simulink model "obstacle"  (R2017a)
settings: Solver=VariableStepAuto  StartTime=0.0  StopTime=10  FixedStep=0.05  RelTol=1e-3
values from neighbouring files (symbols this model uses):
  distance_of_CG = vehical_length/2    (= 0.1825)    [init.m]
  o_x1 = 3    [init.m]
  o_x2 = 5    [init.m]
  o_y1 = 3.3    [init.m]
  o_y2 = 4.7    [init.m]
  psi_init = deg2rad(45)    [init.m]
  x_init = 0    [init.m]
  y_init = 0.2    [init.m]
undefined symbols (not defined in the file or in its folder): theta, x0, y0
undefined symbols (not defined in the file): vehical_length
libraries: simulink_extras x2, simulink x1
settings Model: SnapshotInterval=1  Creator=dell  LastModifiedBy=dell
settings DebuggingCC: InheritedTsInSrcMsg=error

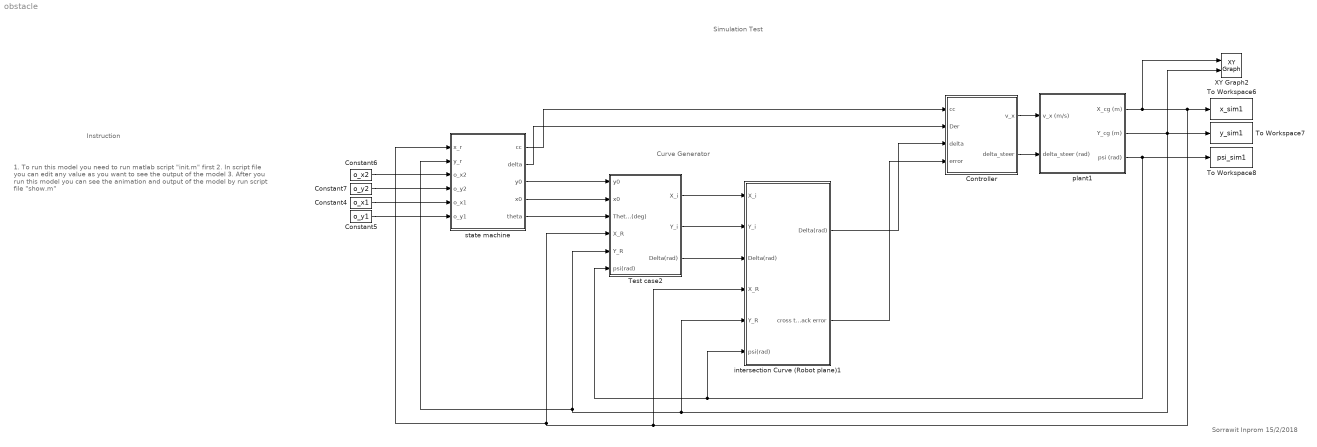
== system obstacle ==
  note: Simulation Test
  note: Sorrawit Inprom
      | 15/2/2018
  note: Curve Generator
  note: Instruction
  note: 1. To run this model you need to run matlab script "init.m" first
      |
      | 2. In script file you can edit any value as you want to see the output of the model
      |
      | 3. After you run this model you can see the animation and output of the model by run script file "show.m"
  Constant4 : Constant  Value=o_x1
  Constant5 : Constant  Value=o_y1
  Constant6 : Constant  Value=o_x2
  Constant7 : Constant  Value=o_y2
  Controller : Subsystem
  Test case2 : Subsystem
  To Workspace6 : ToWorkspace  VariableName=x_sim1  SaveFormat=Timeseries  SampleTime=-1
  To Workspace7 : ToWorkspace  VariableName=y_sim1  SaveFormat=Timeseries  SampleTime=-1
  To Workspace8 : ToWorkspace  VariableName=psi_sim1  SaveFormat=Timeseries  SampleTime=-1
  XY Graph2 : simulink/Sinks/XY Graph  xmin=0  xmax=10  ymin=-1  ymax=10  st=-1
  intersection Curve (Robot plane)1 : Subsystem
  plant1 : Subsystem  mask{vehicle_length=vehical_length, distance_of_CG=distance_of_CG}
      mask prompts: vehicle_length "length"; distance_of_CG "CG"
  state machine : Stateflow chart  TreatAsAtomicUnit=on
  wires:
  state machine/3(y0) -> Test case2/1(y0)
  state machine/4(x0) -> Test case2/2(x0)
  state machine/5(theta) -> Test case2/3(Theta(deg))
  Test case2/1(X_i) -> intersection Curve (Robot plane)1/1(X_i)
  Test case2/2(Y_i) -> intersection Curve (Robot plane)1/2(Y_i)
  Test case2/3("Delta(rad) ") -> intersection Curve (Robot plane)1/3(Delta(rad))
  intersection Curve (Robot plane)1/1("Delta(rad) ") -> Controller/3(delta)
  intersection Curve (Robot plane)1/2(cross track error) -> Controller/4(error)
  Controller/2(delta_steer) -> plant1/2(delta_steer (rad))
  Controller/1(v_x) -> plant1/1(v_x (m/s))
  state machine/1(cc) -> Controller/1(cc)
  state machine/2(delta) -> Controller/2(Der)
  plant1/1(X_cg (m)) -> To Workspace6/1, intersection Curve (Robot plane)1/4(X_R), state machine/1(x_r), Test case2/4(X_R), XY Graph2/1
  plant1/2(Y_cg (m)) -> intersection Curve (Robot plane)1/5(Y_R), state machine/2(y_r), Test case2/5(Y_R), To Workspace7/1, XY Graph2/2
  plant1/3(psi (rad)) -> intersection Curve (Robot plane)1/6(psi(rad)), Test case2/6(psi(rad)), To Workspace8/1
  Constant6/1 -> state machine/3(o_x2)
  Constant7/1 -> state machine/4(o_y2)
  Constant4/1 -> state machine/5(o_x1)
  Constant5/1 -> state machine/6(o_y1)

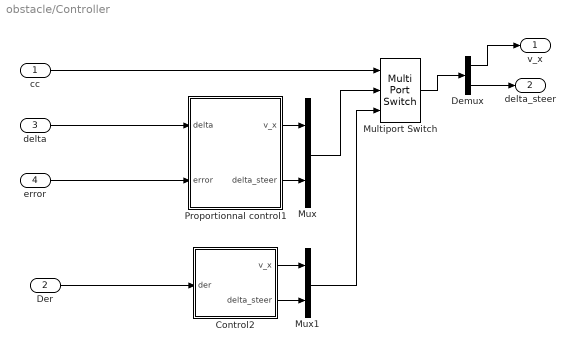
== system obstacle/Controller ==
  cc : Inport
  Der : Inport  Port=2
  delta : Inport  Port=3
  error : Inport  Port=4
  Control2 : Subsystem
  Demux : Demux  Outputs=2
  Multiport Switch : MultiPortSwitch  Inputs=2  DiagnosticForDefault=None
  Mux : Mux  Inputs=2
  Mux1 : Mux  Inputs=2
  Proportionnal control1 : Subsystem
  v_x : Outport
  delta_steer : Outport  Port=2
  wires:
  Multiport Switch/1 -> Demux/1
  Proportionnal control1/2(delta_steer) -> Mux/2
  Mux/1 -> Multiport Switch/2
  Demux/1 -> v_x/1
  Control2/1(v_x) -> Mux1/1
  error/1 -> Proportionnal control1/2(error)
  Der/1 -> Control2/1(der)
  delta/1 -> Proportionnal control1/1(delta)
  Mux1/1 -> Multiport Switch/3
  Control2/2(delta_steer) -> Mux1/2
  cc/1 -> Multiport Switch/1
  Proportionnal control1/1(v_x) -> Mux/1
  Demux/2 -> delta_steer/1

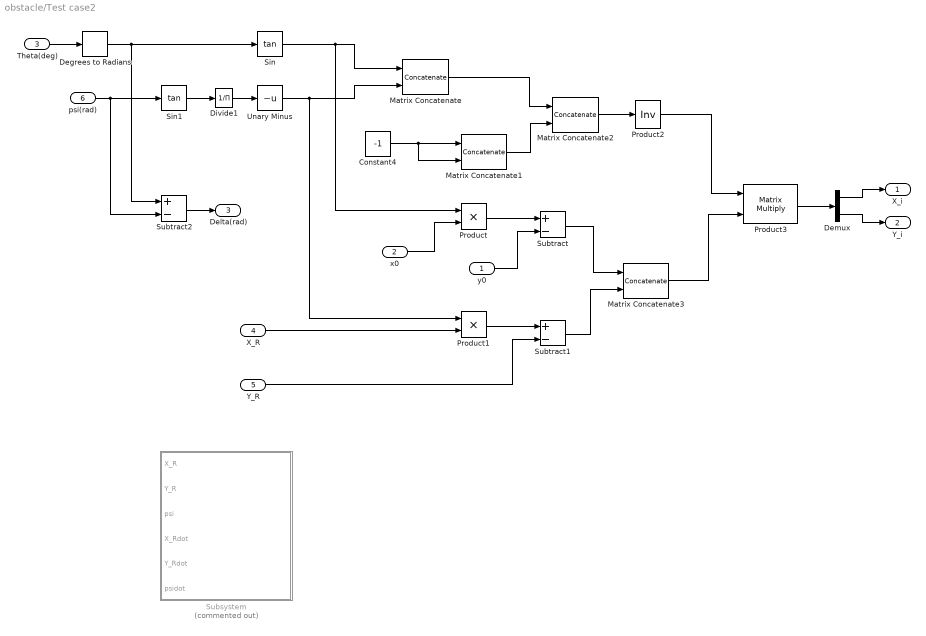
== system obstacle/Test case2 ==
  y0 : Inport
  x0 : Inport  Port=2
  Theta(deg) : Inport  Port=3
  X_R : Inport  Port=4
  Y_R : Inport  Port=5
  psi(rad) : Inport  Port=6
  Constant4 : Constant  Value=-1
  Degrees to Radians : simulink_extras/Transformations/Degrees to Radians
  Demux : Demux  Outputs=2
  Divide1 : Product  Inputs=/
  Matrix Concatenate : Concatenate  Mode=Multidimensional array
  Matrix Concatenate1 : Concatenate  Mode=Multidimensional array
  Matrix Concatenate2 : Concatenate  Mode=Multidimensional array  ConcatenateDimension=2
  Matrix Concatenate3 : Concatenate  Mode=Multidimensional array
  Product : Product
  Product1 : Product
  Product2 : Product  Inputs=/  Multiplication=Matrix(*)
  Product3 : Product  Multiplication=Matrix(*)
  Sin : Trigonometry  Operator=tan
  Sin1 : Trigonometry  Operator=tan
  Subsystem : Subsystem  Commented=on
  Subtract : Sum  Inputs=+-
  Subtract1 : Sum  Inputs=+-
  Subtract2 : Sum  Inputs=+-
  Unary Minus : UnaryMinus
  X_i : Outport
  Y_i : Outport  Port=2
  "Delta(rad) " : Outport  Port=3
  wires:
  Matrix Concatenate2/1 -> Product2/1
  X_R/1 -> Product1/2
  Demux/2 -> Y_i/1
  Matrix Concatenate3/1 -> Product3/2
  Divide1/1 -> Unary Minus/1
  Sin1/1 -> Divide1/1
  y0/1 -> Subtract/2
  x0/1 -> Product/2
  Demux/1 -> X_i/1
  Unary Minus/1 -> Product1/1, Matrix Concatenate/2
  Subtract/1 -> Matrix Concatenate3/1
  Y_R/1 -> Subtract1/2
  Product/1 -> Subtract/1
  Product1/1 -> Subtract1/1
  Subtract1/1 -> Matrix Concatenate3/2
  psi(rad)/1 -> Sin1/1, Subtract2/2
  Constant4/1 -> Matrix Concatenate1/2, Matrix Concatenate1/1
  Matrix Concatenate1/1 -> Matrix Concatenate2/2
  Product2/1 -> Product3/1
  Sin/1 -> Product/1, Matrix Concatenate/1
  Theta(deg)/1 -> Degrees to Radians/1
  Product3/1 -> Demux/1
  Subtract2/1 -> "Delta(rad) "/1
  Matrix Concatenate/1 -> Matrix Concatenate2/1
  Degrees to Radians/1 -> Sin/1, Subtract2/1

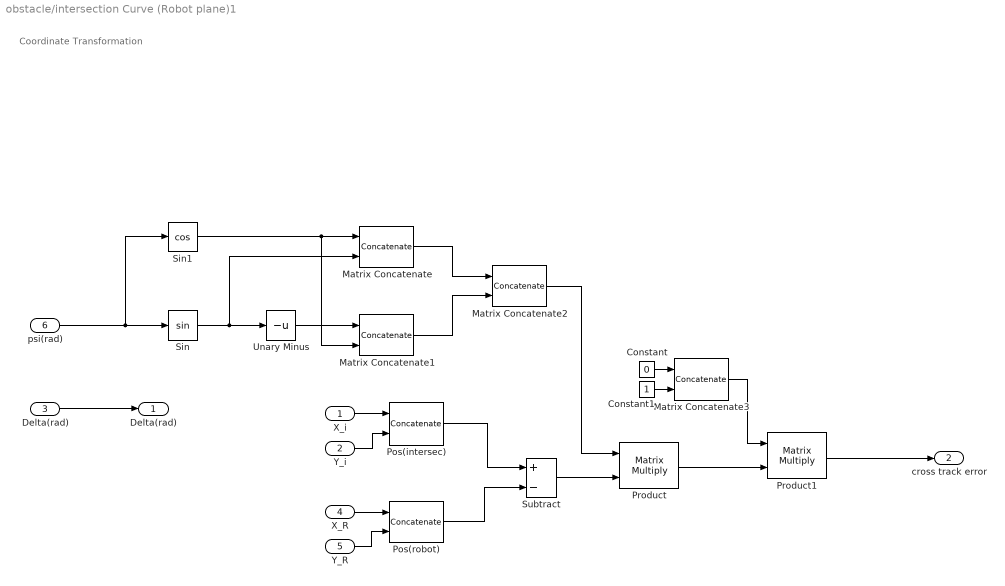
== system obstacle/intersection Curve (Robot plane)1 ==
  note: Coordinate Transformation
  X_i : Inport
  Y_i : Inport  Port=2
  Delta(rad) : Inport  Port=3
  X_R : Inport  Port=4
  Y_R : Inport  Port=5
  psi(rad) : Inport  Port=6
  Constant : Constant  Value=0
  Constant1 : Constant
  Matrix Concatenate : Concatenate  Mode=Multidimensional array  ConcatenateDimension=2
  Matrix Concatenate1 : Concatenate  Mode=Multidimensional array  ConcatenateDimension=2
  Matrix Concatenate2 : Concatenate  Mode=Multidimensional array
  Matrix Concatenate3 : Concatenate  Mode=Multidimensional array  ConcatenateDimension=2
  "Pos(intersec) " : Concatenate  Mode=Multidimensional array
  Pos(robot) : Concatenate  Mode=Multidimensional array
  Product : Product  Multiplication=Matrix(*)
  Product1 : Product  Multiplication=Matrix(*)
  Sin : Trigonometry
  Sin1 : Trigonometry  Operator=cos
  Subtract : Sum  Inputs=+-
  Unary Minus : UnaryMinus
  "Delta(rad) " : Outport
  cross track error : Outport  Port=2
  wires:
  psi(rad)/1 -> Sin1/1, Sin/1
  Matrix Concatenate2/1 -> Product/1
  X_i/1 -> "Pos(intersec) "/1
  Y_i/1 -> "Pos(intersec) "/2
  Subtract/1 -> Product/2
  "Pos(intersec) "/1 -> Subtract/1
  Pos(robot)/1 -> Subtract/2
  Unary Minus/1 -> Matrix Concatenate1/1
  Y_R/1 -> Pos(robot)/2
  X_R/1 -> Pos(robot)/1
  Matrix Concatenate1/1 -> Matrix Concatenate2/2
  Sin1/1 -> Matrix Concatenate/1, Matrix Concatenate1/2
  Matrix Concatenate/1 -> Matrix Concatenate2/1
  Sin/1 -> Matrix Concatenate/2, Unary Minus/1
  Delta(rad)/1 -> "Delta(rad) "/1
  Product/1 -> Product1/2
  Constant/1 -> Matrix Concatenate3/1
  Constant1/1 -> Matrix Concatenate3/2
  Matrix Concatenate3/1 -> Product1/1
  Product1/1 -> cross track error/1

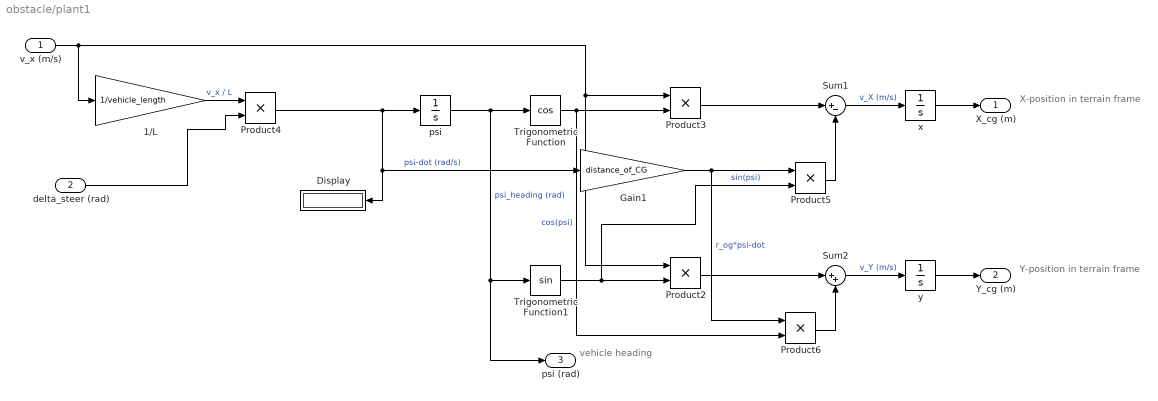
== system obstacle/plant1 ==
  note: vehicle
      | heading
  note: X-position in
      | terrain frame
  note: Y-position in
      | terrain frame
  v_x (m/s) : Inport
  delta_steer (rad) : Inport  Port=2
  1/L : Gain  Gain=1/vehicle_length
  Display : Display
  Gain1 : Gain  Gain=distance_of_CG
  Product{2..6} (5 alike) : Product  RndMeth=Zero
  Sum1 : Sum  Inputs=|+-
  Sum2 : Sum  Inputs=|++
  Trigonometric Function : Trigonometry  Operator=cos
  Trigonometric Function1 : Trigonometry
  psi : Integrator  InitialCondition=psi_init
  x : Integrator  InitialCondition=x_init
  y : Integrator  InitialCondition=y_init
  X_cg (m) : Outport
  Y_cg (m) : Outport  Port=2
  psi (rad) : Outport  Port=3
  wires:
  psi/1 -> Trigonometric Function/1, psi (rad)/1, Trigonometric Function1/1  "psi_heading (rad)"
  x/1 -> X_cg (m)/1
  Trigonometric Function/1 -> Product6/2, Product3/2  "cos(psi)"
  Product4/1 -> Gain1/1, Display/1, psi/1  "psi-dot (rad/s)"
  Sum2/1 -> y/1  "v_Y (m/s)"
  Product6/1 -> Sum2/2
  Product3/1 -> Sum1/1
  y/1 -> Y_cg (m)/1
  Trigonometric Function1/1 -> Product2/2, Product5/2  "sin(psi)"
  Gain1/1 -> Product5/1, Product6/1  "r_og*psi-dot"
  1/L/1 -> Product4/1  "v_x / L"
  Product2/1 -> Sum2/1
  v_x (m/s)/1 -> Product2/1, Product3/1, 1/L/1
  Product5/1 -> Sum1/2
  Sum1/1 -> x/1  "v_X (m/s)"
  delta_steer (rad)/1 -> Product4/2

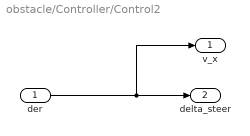
== system obstacle/Controller/Control2 ==
  der : Inport
  v_x : Outport
  delta_steer : Outport  Port=2
  wires:
  der/1 -> v_x/1, delta_steer/1

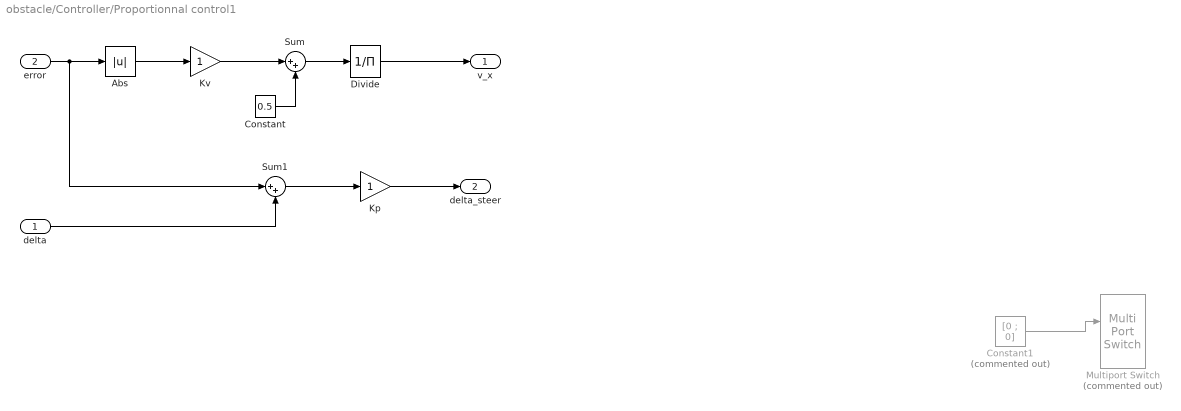
== system obstacle/Controller/Proportionnal control1 ==
  delta : Inport
  error : Inport  Port=2
  Abs : Abs
  Constant : Constant  Value=0.5
  Constant1 : Constant  Commented=on  Value=[0 ; 0]
  Divide : Product  Inputs=/
  Kp : Gain
  Kv : Gain
  Multiport Switch : MultiPortSwitch  Commented=on  DataPortOrder=Zero-based contiguous  Inputs=2  DataPortForDefault=Additional data port
  Sum : Sum  Inputs=|++
  Sum1 : Sum  Inputs=|++
  v_x : Outport  SampleTime=0.1
  delta_steer : Outport  Port=2  SampleTime=0.05
  wires:
  Constant/1 -> Sum/2
  Sum/1 -> Divide/1
  Constant1/1 -> Multiport Switch/2
  Divide/1 -> v_x/1
  Abs/1 -> Kv/1
  Kv/1 -> Sum/1
  Kp/1 -> delta_steer/1
  delta/1 -> Sum1/2
  error/1 -> Sum1/1, Abs/1
  Sum1/1 -> Kp/1

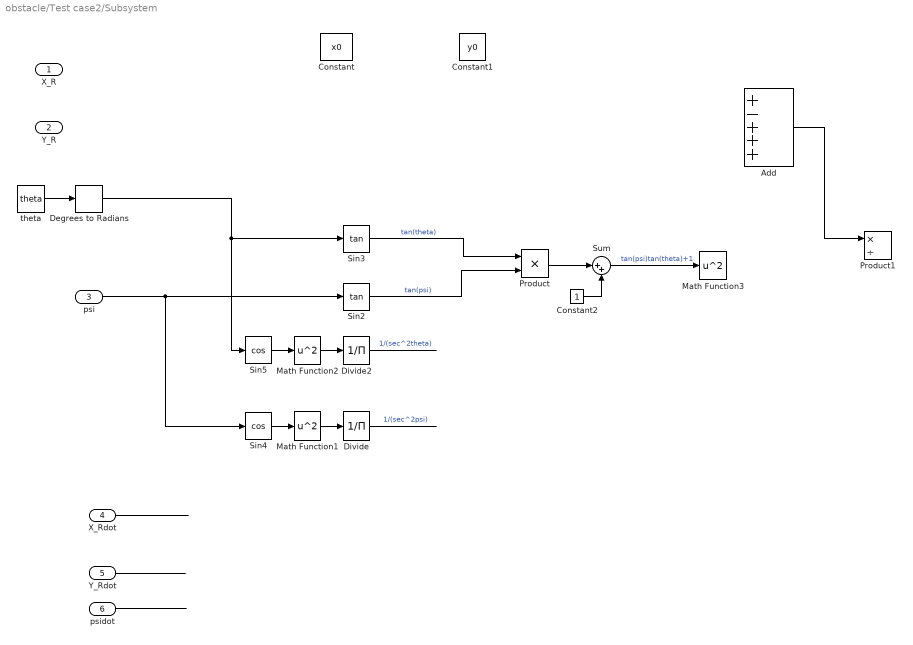
== system obstacle/Test case2/Subsystem ==
  X_R : Inport
  "Y_R " : Inport  Port=2
  psi : Inport  Port=3
  X_Rdot : Inport  Port=4
  Y_Rdot : Inport  Port=5
  psidot : Inport  Port=6
  Add : Sum  Inputs=+-+++
  Constant : Constant  Value=x0
  Constant1 : Constant  Value=y0
  Constant2 : Constant
  Degrees to Radians : simulink_extras/Transformations/Degrees to Radians
  Divide : Product  Inputs=/
  Divide2 : Product  Inputs=/
  Math Function1 : Math  Operator=square  SaturateOnIntegerOverflow=on
  Math Function2 : Math  Operator=square  SaturateOnIntegerOverflow=on
  Math Function3 : Math  Operator=square  SaturateOnIntegerOverflow=on
  Product : Product
  Product1 : Product  Inputs=*/
  Sin2 : Trigonometry  Operator=tan
  Sin3 : Trigonometry  Operator=tan
  Sin4 : Trigonometry  Operator=cos
  Sin5 : Trigonometry  Operator=cos
  Sum : Sum  Inputs=|++
  theta : Constant  Value=theta
  wires:
  Sin3/1 -> Product/1  "tan(theta)"
  Sin4/1 -> Math Function1/1
  Math Function1/1 -> Divide/1
  Divide/1 -> ?  "1/(sec^2psi)"
  X_Rdot/1 -> ?
  Y_Rdot/1 -> ?
  psidot/1 -> ?
  Math Function2/1 -> Divide2/1
  Sin5/1 -> Math Function2/1
  Divide2/1 -> ?  "1/(sec^2theta)"
  psi/1 -> Sin4/1, Sin2/1
  Sin2/1 -> Product/2  "tan(psi)"
  Degrees to Radians/1 -> Sin5/1, Sin3/1
  theta/1 -> Degrees to Radians/1
  Product/1 -> Sum/1
  Constant2/1 -> Sum/2
  Sum/1 -> Math Function3/1  "tan(psi)tan(theta)+1"
  Add/1 -> Product1/1

== stateflow chart obstacle/state machine ==
  state Initial
    entry:
    delta = 0;
    dist1 = 10;
    dist2 = 10;
  state turn_right [commented out]
    entry:
    cc = 2;
    delta = deg2rad(-15);
  state right_lane
    entry:
    x0 = 0;
    y0 = -0.3;
    theta = 45;
    during:
    dist2 = sqrt((o_x2 - x_r)^2 + (o_y2 - y_r)^2);
  state left_lane
    entry:
    x0 = 0;
    y0 = 0.3;
    theta = 45;
    cc = 1;
    during:
    dist1 = sqrt((o_x1 - x_r)^2 + (o_y1 - y_r)^2);
  state turn_left [commented out]
    entry:
    cc = 2;
    delta = deg2rad(15);
  state stop
    entry:
    cc = 2;
    delta = 0;
  state left_lane1
    entry:
    x0 = 0;
    y0 = 0.3;
    theta = 45;
  (default) -> Initial
  left_lane -> right_lane : [dist1 <= 1.5]
  Initial -> left_lane
  turn_right -> right_lane [commented out] : [x_r >= 2.8]
  left_lane -> turn_right [commented out] : [x_r >= 2.5]
  right_lane -> turn_left [commented out] : [x_r >= 4.5]
  turn_left -> left_lane [commented out] : [x_r >= 4.8 ]
  right_lane -> left_lane1 : [dist2 <= 1.5]
  left_lane1 -> stop : [x_r >= 7.8]
  data: cc output; x_r input; y_r input; delta output; y0 output; x0 output; theta output; o_x2 input; o_y2 input; o_x1 input; o_y1 input; dist2 local; dist1 local
